simulink model "ModifiedHVDC"  (R2024b)
settings: Solver=ode3  StartTime=0.0  StopTime=2.5  FixedStep=7.4074074074074075E-6  RelTol=1e-3  AbsTol=1e-2
InitFcn:
  | Fnom = 50;        % Hz
  | 
  | Fc = 27*Fnom;   % (Hz)
  | Ts_Power = 1/(Fc*100);
  | Ts_Control = Ts_Power*10;
values from neighbouring files (symbols this model uses):
  C_per_km = 2.3100e-007    (= 2.31e-07)    [Parameters.m]
  L_per_km = 1.5900e-004    (= 0.000159)    [Parameters.m]
  L_total = 75    [Parameters.m]
  R_per_km = 1.3900e-002    (= 0.0139)    [Parameters.m]
  x_fault = 13    [Parameters.m]
undefined symbols (not defined in the file or in its folder): D1, Delta, DiscIntNeverNeededParam, magnitude
libraries: spsSecondOrderFilterLib x20, spsSeriesRLCBranchLib x14, spsMeanVariableFrequencyLib x12, spsabctoAlphaBetaZeroLib x8, spsThreePhaseVIMeasurementLib x6, spsAlphaBetaZerotodq0Lib x6, spsPiSectionLineLib x4, spsCurrentMeasurementLib x4, spsThreePhaseHarmonicFilterLib x4, spsVoltageMeasurementLib x4, spsFirstOrderFilterLib x4, spsGroundLib x3
(part 4 of 5)

== system ModifiedHVDC/VSC Controller Station 2/Discrete VSC Controller /Outer Active-Reactive Power and Voltage Loop/Reactive_Power_Control ==
  note: Output is added to the regulator reference
      |  in order to maintain the AC voltage within
      |  minimum and maximum limits
  note: Reactive Power Control
  enable_control : Inport
  Qref : Inport  Port=2
  Q_meas : Inport  Port=3
  U_meas : Inport  Port=4
  "AC Voltage Control Override " : Subsystem  mask(Regulator with override functionality){max_in=U_max, min_in=U_min, Ki=Ki_rpc_vco, Kp=Kp_rpc_vco, IC_i=0, max_out_lim=max_rpc_vco, min_out_lim=min_rpc_vco, Ts=Ts_Control}
      mask prompts: max_in "Input upper range (pu):"; min_in "Input lower range (pu):"; Ki "Integrator gain (pu/s):"; Kp "Proportional gain:"; IC_i "Integrator initial condition (pu):"; max_out_lim "Output maximum limit (pu):"; min_out_lim "Output minimum limit (pu):"; Ts "Sample time: (s)"
      mask Display: disp('Override \nRegulator')
  Add : Sum
  Freeze_integrator : Subsystem
  Gain : Gain  Gain=-1
  Int_regulator (type 1) : Subsystem  mask(Feed forward integral regulator with anti-windup and freeze - type 1){max_i=max_i_rpc, min_i=min_i_rpc, Ki=Ki_rpc, IC_i=0, Kf=1.0, max_out=Q_max, min_out=Q_min, Ts=Ts_Control}
      mask prompts: max_i "Integrator maximum  limit (pu):"; min_i "Integrator minimum  limit (pu):"; Ki "Integrator gain (pu/s):"; IC_i "Integrator initial condition (pu):"; Kf "Feadback gain :"; max_out "Output maximum limit (pu):"; min_out "Output minimum limit (pu):"; Ts "Sample time: (s)"
      mask help:
      | The reference (input 1) is fed forward to the output. The integrator compensates for any steady-state error between the desired (input 1) and the measured value input 2). The error signal (input 1 - input 2) is integrated with dynamic limits (Integrator min and max limits). The integration can be frozen (stopped) when input 3 is TRUE.
      | A back-calculation anti-windup method discharges the integrator on block saturation (output min and max limits) using a feedback loop having a gain coefficient.
      mask Display: disp('Integral \n(Type 1)')
  Saturation : Saturate  UpperLimit=Q_max  LowerLimit=Q_min
      settings: AttributesFormatString=Min=%<LowerLimit>\nMax=%<UpperLimit>
  Qref_rpc : Outport  VectorParamsAs1DForOutWhenUnconnected=off
  wires:
  Gain/1 -> Add/1
  Add/1 -> Saturation/1
  "AC Voltage Control Override "/1(Out) -> Add/2
  Int_regulator (type 1)/1(Out) -> Gain/1
  U_meas/1 -> Freeze_integrator/1(U_meas), "AC Voltage Control Override "/1(In)
  Saturation/1 -> Qref_rpc/1
  Qref/1 -> Int_regulator (type 1)/1(Ord)
  Q_meas/1 -> Int_regulator (type 1)/2(Meas)
  enable_control/1 -> Int_regulator (type 1)/Enable, "AC Voltage Control Override "/Enable
  Freeze_integrator/1(Freeze) -> Int_regulator (type 1)/3(freeze)

== system ModifiedHVDC/VSC Controller Station 2/Discrete VSC Controller /PLL/Discrete PI Controller ==
  note: Pierre Giroux, Gilbert Sybille
      | Power System Simulation Laboratory
      | IREQ, Hydro-Quebc
  note: Discrete PID Controller
  Error : Inport  SampleTime=Ts
  Discrete-Time Integrator : DiscreteIntegrator  InitialCondition=Init  SampleTime=Ts  LimitOutput=on  UpperSaturationLimit=UpperLimit  LowerSaturationLimit=LowerLimit  ICPrevOutput=DiscIntNeverNeededParam  ICPrevScaledInput=DiscIntNeverNeededParam
  Kp4 : Gain  Gain=Kp  SaturateOnIntegerOverflow=on  SampleTime=Ts  OutDataTypeStr=Inherit: Same as input  ParamDataTypeStr=Inherit: Same as input
  Kp5 : Gain  Gain=Ki  SaturateOnIntegerOverflow=on  SampleTime=Ts  OutDataTypeStr=Inherit: Same as input  ParamDataTypeStr=Inherit: Same as input
  Saturation2 : Saturate  UpperLimit=UpperLimit  LowerLimit=LowerLimit  SampleTime=Ts
  Sum6 : Sum  InputSameDT=on  SaturateOnIntegerOverflow=on  SampleTime=Ts  OutDataTypeStr=Inherit: Same as first input
  Zero-Order Hold : ZeroOrderHold  SampleTime=Ts
  Out : Outport  SampleTime=Ts  InitialOutput=0  VectorParamsAs1DForOutWhenUnconnected=off
  wires:
  Error/1 -> Kp4/1, Kp5/1
  Sum6/1 -> Saturation2/1
  Kp5/1 -> Discrete-Time Integrator/1
  Kp4/1 -> Zero-Order Hold/1
  Discrete-Time Integrator/1 -> Sum6/2
  Saturation2/1 -> Out/1
  Zero-Order Hold/1 -> Sum6/1

== system ModifiedHVDC/VSC Controller Station 2/Discrete VSC Controller /PLL/Discrete Rate Limiter ==
  note: Delta(u)
  note: Beat Ronner
      | ABB Industrie AG
      | Turgi, Switzerland
  In : Inport
  Saturation : Saturate  UpperLimit=UpperLimit  LowerLimit=LowerLimit
  Sum : Sum  Inputs=|++  InputSameDT=on  SaturateOnIntegerOverflow=on  OutDataTypeStr=Inherit: Same as first input
  Sum1 : Sum  Inputs=|+-  InputSameDT=on  SaturateOnIntegerOverflow=on  OutDataTypeStr=Inherit: Same as first input
  Unit Delay : UnitDelay  InitialCondition=Vinit  SampleTime=Ts  HasFrameUpgradeWarning=on
  Out : Outport  VectorParamsAs1DForOutWhenUnconnected=off
  wires:
  In/1 -> Sum1/1  "u"
  Sum1/1 -> Saturation/1
  Saturation/1 -> Sum/1  "Delta(u)_limit"
  Sum/1 -> Out/1, Unit Delay/1  "y"
  Unit Delay/1 -> Sum1/2, Sum/2  "y-1"

== system ModifiedHVDC/VSC Controller Station 2/Discrete VSC Controller /Signal Calculations/Active_Power ==
  note: Active Power Calculation
  U_AB : Inport
  I_AB : Inport  Port=2
  Demux : Demux  Outputs=2
      settings: DisplayOption=none
  Demux1 : Demux  Outputs=2
      settings: DisplayOption=none
  Product : Product  SaturateOnIntegerOverflow=on  OutDataTypeStr=Inherit: Same as first input
  Product1 : Product  SaturateOnIntegerOverflow=on  OutDataTypeStr=Inherit: Same as first input
  Sum : Sum  SaturateOnIntegerOverflow=on
  Ppcc : Outport  VectorParamsAs1DForOutWhenUnconnected=off
  wires:
  U_AB/1 -> Demux/1
  I_AB/1 -> Demux1/1
  Demux/1 -> Product/1
  Demux1/1 -> Product/2
  Demux/2 -> Product1/1
  Demux1/2 -> Product1/2
  Product/1 -> Sum/1
  Product1/1 -> Sum/2
  Sum/1 -> Ppcc/1

== system ModifiedHVDC/VSC Controller Station 2/Discrete VSC Controller /Signal Calculations/DC_Current ==
  note: DC Current Calculation
  Idc_p : Inport
  Idc_n : Inport  Port=2
  Gain : Gain  Gain=0.5  SaturateOnIntegerOverflow=on  OutDataTypeStr=Inherit: Same as input  ParamDataTypeStr=Inherit: Same as input
  Sum : Sum  Inputs=+-  SaturateOnIntegerOverflow=on
  Idc_meas : Outport  VectorParamsAs1DForOutWhenUnconnected=off
  wires:
  Gain/1 -> Idc_meas/1
  Sum/1 -> Gain/1
  Idc_n/1 -> Sum/2
  Idc_p/1 -> Sum/1

== system ModifiedHVDC/VSC Controller Station 2/Discrete VSC Controller /Signal Calculations/DC_Voltage ==
  note: DC Voltage Calculation
  Udc_p : Inport
  Udc_n : Inport  Port=2
  Gain : Gain  Gain=0.5  SaturateOnIntegerOverflow=on  OutDataTypeStr=Inherit: Same as input  ParamDataTypeStr=Inherit: Same as input
  Sum : Sum  Inputs=+-  SaturateOnIntegerOverflow=on
  Udc_meas : Outport  VectorParamsAs1DForOutWhenUnconnected=off
  wires:
  Udc_p/1 -> Sum/1
  Sum/1 -> Gain/1
  Gain/1 -> Udc_meas/1
  Udc_n/1 -> Sum/2

== system ModifiedHVDC/VSC Controller Station 2/Discrete VSC Controller /Signal Calculations/Filter_Bus_Voltage ==
  note: Filter Bus Voltage Calculation
  Uf_AB : Inport
  Math Function : Math  Operator=magnitude^2  SignedPower=on
  Math Function1 : Math  Operator=sqrt  SignedPower=on
  Sum : Sum  Inputs=+  SaturateOnIntegerOverflow=on
  Uf_meas : Outport  VectorParamsAs1DForOutWhenUnconnected=off
  wires:
  Math Function1/1 -> Uf_meas/1
  Sum/1 -> Math Function1/1
  Math Function/1 -> Sum/1
  Uf_AB/1 -> Math Function/1

== system ModifiedHVDC/VSC Controller Station 2/Discrete VSC Controller /Signal Calculations/Modulation_Index ==
  note: Modulation Index Calculation
  Vref_lim_AB : Inport
  Udc_meas : Inport  Port=2
  Gain1 : Gain  Gain=k_pu2nom_Vdc  SaturateOnIntegerOverflow=on  OutDataTypeStr=Inherit: Same as input  ParamDataTypeStr=Inherit: Same as input
  MAX:10 MIN: 0 : Saturate  UpperLimit=10  LowerLimit=0
  Math Function1 : Math  Operator=magnitude^2  SignedPower=on
  Math Function2 : Math  Operator=sqrt  SignedPower=on
  Product : Product  Inputs=*/  SaturateOnIntegerOverflow=on  OutDataTypeStr=Inherit: Same as first input
  Saturation : Saturate  UpperLimit=1e6  LowerLimit=1e-6
  Sum : Sum  Inputs=+  SaturateOnIntegerOverflow=on
  Mod_index : Outport  VectorParamsAs1DForOutWhenUnconnected=off
  wires:
  Gain1/1 -> Saturation/1
  MAX:10 MIN: 0/1 -> Mod_index/1
  Saturation/1 -> Product/2
  Product/1 -> MAX:10 MIN: 0/1
  Udc_meas/1 -> Gain1/1
  Sum/1 -> Math Function2/1
  Math Function1/1 -> Sum/1
  Math Function2/1 -> Product/1
  Vref_lim_AB/1 -> Math Function1/1

== system ModifiedHVDC/VSC Controller Station 2/Discrete VSC Controller /Signal Calculations/PCC_Voltage ==
  note: Active Power Calculation
  U_AB : Inport
  Math Function : Math  Operator=magnitude^2  SignedPower=on
  Math Function1 : Math  Operator=sqrt  SignedPower=on
  Sum : Sum  Inputs=+  SaturateOnIntegerOverflow=on
  Upcc : Outport  VectorParamsAs1DForOutWhenUnconnected=off
  wires:
  U_AB/1 -> Math Function/1
  Math Function/1 -> Sum/1
  Sum/1 -> Math Function1/1
  Math Function1/1 -> Upcc/1

== system ModifiedHVDC/VSC Controller Station 2/Discrete VSC Controller /Signal Calculations/Reactive_Power ==
  note: Reactive Power Calculation
  U_AB : Inport
  I_AB : Inport  Port=2
  Demux : Demux  Outputs=2
      settings: DisplayOption=none
  Demux1 : Demux  Outputs=2
      settings: DisplayOption=none
  Product : Product  SaturateOnIntegerOverflow=on  OutDataTypeStr=Inherit: Same as first input
  Product1 : Product  SaturateOnIntegerOverflow=on  OutDataTypeStr=Inherit: Same as first input
  Sum : Sum  Inputs=+-  SaturateOnIntegerOverflow=on
  Qpcc : Outport  VectorParamsAs1DForOutWhenUnconnected=off
  wires:
  Sum/1 -> Qpcc/1
  Product1/1 -> Sum/2
  Product/1 -> Sum/1
  I_AB/1 -> Demux1/1
  U_AB/1 -> Demux/1
  Demux/2 -> Product/2
  Demux1/1 -> Product/1
  Demux/1 -> Product1/1
  Demux1/2 -> Product1/2

== system ModifiedHVDC/VSC Controller Station 1/Discrete VSC Controller /Clark Transformations/CLARK  with Rotating reference/CLARK ==
  note: CLARK transformation
  abc : Inport
  Enable (held) : EnablePort  PropagateVarSize=During execution
  abc to Alpha-Beta-Zero : spsabctoAlphaBetaZeroLib/abc to Alpha-Beta-Zero
  AB0 : Outport  VectorParamsAs1DForOutWhenUnconnected=off
  wires:
  abc to Alpha-Beta-Zero/1 -> AB0/1
  abc/1 -> abc to Alpha-Beta-Zero/1

== system ModifiedHVDC/VSC Controller Station 1/Discrete VSC Controller /Clark Transformations/CLARK  with Rotating reference/CLARK_lag ==
  note: CLARK transformation - YD1
  abc : Inport
  Enable : EnablePort  PropagateVarSize=During execution
  Fcn1 : Fcn  Expr=(-u[1] - u[3] + 2*u[2] )/3
  Fcn2 : Fcn  Expr=(u[1]-u[3])/sqrt(3)
  Fcn3 : Fcn  Expr=0
  Mux : Mux  Inputs=3
  AB0 : Outport  VectorParamsAs1DForOutWhenUnconnected=off
  wires:
  Fcn2/1 -> Mux/1
  abc/1 -> Fcn1/1, Fcn3/1, Fcn2/1
  Fcn1/1 -> Mux/2
  Fcn3/1 -> Mux/3
  Mux/1 -> AB0/1

== system ModifiedHVDC/VSC Controller Station 1/Discrete VSC Controller /Clark Transformations/CLARK  with Rotating reference/CLARK_lead ==
  note: CLARK transformation - YD11
  abc : Inport
  Enable : EnablePort  PropagateVarSize=During execution
  Fcn1 : Fcn  Expr=(u[1] + u[2] - 2*u[3] )/3
  Fcn2 : Fcn  Expr=(u[1]-u[2])/sqrt(3)
  Fcn3 : Fcn  Expr=0
  Mux : Mux  Inputs=3
  AB0 : Outport  VectorParamsAs1DForOutWhenUnconnected=off
  wires:
  Mux/1 -> AB0/1
  Fcn3/1 -> Mux/3
  Fcn1/1 -> Mux/2
  abc/1 -> Fcn2/1, Fcn3/1, Fcn1/1
  Fcn2/1 -> Mux/1

== system ModifiedHVDC/VSC Controller Station 1/Discrete VSC Controller /Clark Transformations/CLARK  with Rotating reference1/CLARK ==
  note: CLARK transformation
  abc : Inport
  Enable (held) : EnablePort  PropagateVarSize=During execution
  abc to Alpha-Beta-Zero : spsabctoAlphaBetaZeroLib/abc to Alpha-Beta-Zero
  AB0 : Outport  VectorParamsAs1DForOutWhenUnconnected=off
  wires:
  abc to Alpha-Beta-Zero/1 -> AB0/1
  abc/1 -> abc to Alpha-Beta-Zero/1

== system ModifiedHVDC/VSC Controller Station 1/Discrete VSC Controller /Clark Transformations/CLARK  with Rotating reference1/CLARK_lag ==
  note: CLARK transformation - YD1
  abc : Inport
  Enable : EnablePort  PropagateVarSize=During execution
  Fcn1 : Fcn  Expr=(-u[1] - u[3] + 2*u[2] )/3
  Fcn2 : Fcn  Expr=(u[1]-u[3])/sqrt(3)
  Fcn3 : Fcn  Expr=0
  Mux : Mux  Inputs=3
  AB0 : Outport  VectorParamsAs1DForOutWhenUnconnected=off
  wires:
  Fcn2/1 -> Mux/1
  abc/1 -> Fcn1/1, Fcn3/1, Fcn2/1
  Fcn1/1 -> Mux/2
  Fcn3/1 -> Mux/3
  Mux/1 -> AB0/1

== system ModifiedHVDC/VSC Controller Station 1/Discrete VSC Controller /Clark Transformations/CLARK  with Rotating reference1/CLARK_lead ==
  note: CLARK transformation - YD11
  abc : Inport
  Enable : EnablePort  PropagateVarSize=During execution
  Fcn1 : Fcn  Expr=(u[1] + u[2] - 2*u[3] )/3
  Fcn2 : Fcn  Expr=(u[1]-u[2])/sqrt(3)
  Fcn3 : Fcn  Expr=0
  Mux : Mux  Inputs=3
  AB0 : Outport  VectorParamsAs1DForOutWhenUnconnected=off
  wires:
  Mux/1 -> AB0/1
  Fcn3/1 -> Mux/3
  Fcn1/1 -> Mux/2
  abc/1 -> Fcn2/1, Fcn3/1, Fcn1/1
  Fcn2/1 -> Mux/1

== system ModifiedHVDC/VSC Controller Station 1/Discrete VSC Controller /DC Voltage Balance Control/Regulator/PI_regulator (type 2) ==
  note: Regulator PI
      | (Type 2)
  Ord : Inport
  Meas : Inport  Port=2
  Add : Sum
  Add1 : Sum
  Discrete-Time Integrator : DiscreteIntegrator  IntegratorMethod=Integration: Trapezoidal  gainval=Ki  InitialCondition=i_ic  SampleTime=Ts  LimitOutput=on  UpperSaturationLimit=max_i  LowerSaturationLimit=min_i  ICPrevOutput=DiscIntNeverNeededParam  ICPrevScaledInput=DiscIntNeverNeededParam
      settings: AttributesFormatString=Gain=%<gainval>\nMin=%<LowerSaturationLimit>\nMax=%<UpperSaturationLimit>
  Kf : Gain  Gain=Kf
      settings: AttributesFormatString=Gain=%<Gain>
  Kp : Gain  Gain=Kp
      settings: AttributesFormatString=Gain=%<Gain>
  Saturation : Saturate  UpperLimit=max_out  LowerLimit=min_out
      settings: AttributesFormatString=Min=%<LowerLimit>\nMax=%<UpperLimit>
  Subtract : Sum  Inputs=+-
  Sum2 : Sum  Inputs=|+-  SaturateOnIntegerOverflow=on
  Unit Delay : UnitDelay  SampleTime=Ts_Control  HasFrameUpgradeWarning=on
      settings: AttributesFormatString=IC=%<InitialCondition>
  Out : Outport  VectorParamsAs1DForOutWhenUnconnected=off
  wires:
  Kp/1 -> Add1/1
  Sum2/1 -> Kf/1
  Subtract/1 -> Add/1, Kp/1
  Saturation/1 -> Sum2/1, Out/1
  Unit Delay/1 -> Add/2
  Add/1 -> Discrete-Time Integrator/1
  Ord/1 -> Subtract/1
  Kf/1 -> Unit Delay/1
  Add1/1 -> Saturation/1, Sum2/2
  Discrete-Time Integrator/1 -> Add1/2
  Meas/1 -> Subtract/2

== system ModifiedHVDC/VSC Controller Station 1/Discrete VSC Controller /Inner Current Loop/AC_Current_Control/PI_regulator 1 ==
  note: Regulator PI
      | (Type 2)
  Ord : Inport
  Meas : Inport  Port=2
  Add : Sum
  Add1 : Sum
  Discrete-Time Integrator : DiscreteIntegrator  IntegratorMethod=Integration: Trapezoidal  gainval=Ki  InitialCondition=i_ic  SampleTime=Ts  LimitOutput=on  UpperSaturationLimit=max_i  LowerSaturationLimit=min_i  ICPrevOutput=DiscIntNeverNeededParam  ICPrevScaledInput=DiscIntNeverNeededParam
      settings: AttributesFormatString=Gain=%<gainval>\nMin=%<LowerSaturationLimit>\nMax=%<UpperSaturationLimit>
  Kf : Gain  Gain=Kf
      settings: AttributesFormatString=Gain=%<Gain>
  Kp : Gain  Gain=Kp
      settings: AttributesFormatString=Gain=%<Gain>
  Saturation : Saturate  UpperLimit=max_out  LowerLimit=min_out
      settings: AttributesFormatString=Min=%<LowerLimit>\nMax=%<UpperLimit>
  Subtract : Sum  Inputs=+-
  Sum2 : Sum  Inputs=|+-  SaturateOnIntegerOverflow=on
  Unit Delay : UnitDelay  SampleTime=Ts_Control  HasFrameUpgradeWarning=on
      settings: AttributesFormatString=IC=%<InitialCondition>
  Out : Outport  VectorParamsAs1DForOutWhenUnconnected=off
  wires:
  Kp/1 -> Add1/1
  Sum2/1 -> Kf/1
  Subtract/1 -> Add/1, Kp/1
  Saturation/1 -> Sum2/1, Out/1
  Unit Delay/1 -> Add/2
  Add/1 -> Discrete-Time Integrator/1
  Ord/1 -> Subtract/1
  Kf/1 -> Unit Delay/1
  Add1/1 -> Saturation/1, Sum2/2
  Discrete-Time Integrator/1 -> Add1/2
  Meas/1 -> Subtract/2

== system ModifiedHVDC/VSC Controller Station 1/Discrete VSC Controller /Inner Current Loop/AC_Current_Control/PI_regulator 2 ==
  note: Regulator PI
      | (Type 2)
  Ord : Inport
  Meas : Inport  Port=2
  Add : Sum
  Add1 : Sum
  Discrete-Time Integrator : DiscreteIntegrator  IntegratorMethod=Integration: Trapezoidal  gainval=Ki  InitialCondition=i_ic  SampleTime=Ts  LimitOutput=on  UpperSaturationLimit=max_i  LowerSaturationLimit=min_i  ICPrevOutput=DiscIntNeverNeededParam  ICPrevScaledInput=DiscIntNeverNeededParam
      settings: AttributesFormatString=Gain=%<gainval>\nMin=%<LowerSaturationLimit>\nMax=%<UpperSaturationLimit>
  Kf : Gain  Gain=Kf
      settings: AttributesFormatString=Gain=%<Gain>
  Kp : Gain  Gain=Kp
      settings: AttributesFormatString=Gain=%<Gain>
  Saturation : Saturate  UpperLimit=max_out  LowerLimit=min_out
      settings: AttributesFormatString=Min=%<LowerLimit>\nMax=%<UpperLimit>
  Subtract : Sum  Inputs=+-
  Sum2 : Sum  Inputs=|+-  SaturateOnIntegerOverflow=on
  Unit Delay : UnitDelay  SampleTime=Ts_Control  HasFrameUpgradeWarning=on
      settings: AttributesFormatString=IC=%<InitialCondition>
  Out : Outport  VectorParamsAs1DForOutWhenUnconnected=off
  wires:
  Kp/1 -> Add1/1
  Sum2/1 -> Kf/1
  Subtract/1 -> Add/1, Kp/1
  Saturation/1 -> Sum2/1, Out/1
  Unit Delay/1 -> Add/2
  Add/1 -> Discrete-Time Integrator/1
  Ord/1 -> Subtract/1
  Kf/1 -> Unit Delay/1
  Add1/1 -> Saturation/1, Sum2/2
  Discrete-Time Integrator/1 -> Add1/2
  Meas/1 -> Subtract/2

== system ModifiedHVDC/VSC Controller Station 1/Discrete VSC Controller /Outer Active-Reactive Power and Voltage Loop/Active_Power_Control/DC Voltage Control Override ==
  note: Reset states when enabling
  note: Override Regulator
  note: Active when input (In) is outside its range [min_in, max_in] otherwise the output goes back to zero
  In : Inport
  Enable (reset) : EnablePort  StatesWhenEnabling=reset  PropagateVarSize=During execution
  Add : Sum
  Constant1 : Constant  Value=max_in
  Constant2 : Constant  Value=min_in
  Constant3 : Constant  Value=Kp
  Discrete-Time Integrator1 : DiscreteIntegrator  IntegratorMethod=Integration: Trapezoidal  gainval=Ki  InitialCondition=IC_i  SampleTime=Ts  LimitOutput=on  UpperSaturationLimit=0  LowerSaturationLimit=min_out_lim  ICPrevOutput=DiscIntNeverNeededParam  ICPrevScaledInput=DiscIntNeverNeededParam
      settings: AttributesFormatString=Gain=%<gainval>\nMin=%<LowerSaturationLimit>\nMax=%<UpperSaturationLimit>
  Discrete-Time Integrator2 : DiscreteIntegrator  IntegratorMethod=Integration: Trapezoidal  gainval=Ki  InitialCondition=IC_i  SampleTime=Ts  LimitOutput=on  UpperSaturationLimit=max_out_lim  LowerSaturationLimit=0  ICPrevOutput=DiscIntNeverNeededParam  ICPrevScaledInput=DiscIntNeverNeededParam
      settings: AttributesFormatString=Gain=%<gainval>\nMin=%<LowerSaturationLimit>\nMax=%<UpperSaturationLimit>
  Product : Product  RndMeth=Zero
  Saturation : Saturate  UpperLimit=0  LowerLimit=min_out_lim
      settings: AttributesFormatString=Min=%<LowerLimit>\nMax=%<UpperLimit>
  Saturation1 : Saturate  UpperLimit=max_out_lim  LowerLimit=0
      settings: AttributesFormatString=Min=%<LowerLimit>\nMax=%<UpperLimit>
  Saturation2 : Saturate  UpperLimit=max_out_lim  LowerLimit=min_out_lim
      settings: AttributesFormatString=Min=%<LowerLimit>\nMax=%<UpperLimit>
  Subtract : Sum  Inputs=+-
  Subtract1 : Sum  Inputs=-+
  Sum2 : Sum  Inputs=+++  SaturateOnIntegerOverflow=on
  Out : Outport  VectorParamsAs1DForOutWhenUnconnected=off
  wires:
  Constant2/1 -> Subtract1/2
  Constant1/1 -> Subtract/1
  Discrete-Time Integrator2/1 -> Sum2/3  "positive"
  Discrete-Time Integrator1/1 -> Sum2/2  "negative"
  Product/1 -> Sum2/1
  Saturation1/1 -> Add/2
  Saturation/1 -> Add/1
  Add/1 -> Product/2
  Constant3/1 -> Product/1
  In/1 -> Subtract1/1, Subtract/2
  Subtract/1 -> Discrete-Time Integrator1/1, Saturation/1
  Subtract1/1 -> Saturation1/1, Discrete-Time Integrator2/1
  Sum2/1 -> Saturation2/1
  Saturation2/1 -> Out/1

== system ModifiedHVDC/VSC Controller Station 1/Discrete VSC Controller /Outer Active-Reactive Power and Voltage Loop/Active_Power_Control/Freeze_integrator ==
  note: Low AC voltage level
  note: Freeze Integrator
  U_meas : Inport
  Constant8 : Constant  Value=V_level_apc
  Relational Operator : RelationalOperator  Operator=<=  InputSameDT=off
  Freeze : Outport  VectorParamsAs1DForOutWhenUnconnected=off
  wires:
  Constant8/1 -> Relational Operator/2
  Relational Operator/1 -> Freeze/1
  U_meas/1 -> Relational Operator/1

== system ModifiedHVDC/VSC Controller Station 1/Discrete VSC Controller /Outer Active-Reactive Power and Voltage Loop/Active_Power_Control/Int_regulator (type 1) ==
  note: Reset states when enabling
  note: Integral Regulator
      | (Type 1)
  Ord : Inport
  Meas : Inport  Port=2
  freeze : Inport  Port=3
  Enable (Reset) : EnablePort  StatesWhenEnabling=reset  PropagateVarSize=During execution
  Add : Sum
  Add1 : Sum
  Constant7 : Constant  Value=0.0
  Discrete-Time Integrator : DiscreteIntegrator  IntegratorMethod=Integration: Trapezoidal  gainval=Ki  InitialCondition=IC_i  SampleTime=Ts  LimitOutput=on  UpperSaturationLimit=max_i  LowerSaturationLimit=min_i  ICPrevOutput=DiscIntNeverNeededParam  ICPrevScaledInput=DiscIntNeverNeededParam
      settings: AttributesFormatString=Gain=%<gainval>\nMin=%<LowerSaturationLimit>\nMax=%<UpperSaturationLimit>
  Kf : Gain  Gain=Kf
      settings: AttributesFormatString=Gain=%<Gain>
  Saturation : Saturate  UpperLimit=max_out  LowerLimit=min_out
      settings: AttributesFormatString=Min=%<LowerLimit>\nMax=%<UpperLimit>
  Subtract : Sum  Inputs=+-
  Sum2 : Sum  Inputs=|+-  SaturateOnIntegerOverflow=on
  Switch : Switch  Criteria=u2 > Threshold  InputSameDT=off
  Unit Delay : UnitDelay  SampleTime=Ts_Control  HasFrameUpgradeWarning=on
      settings: AttributesFormatString=IC=%<InitialCondition>
  Out : Outport  VectorParamsAs1DForOutWhenUnconnected=off
  wires:
  Kf/1 -> Unit Delay/1
  Subtract/1 -> Switch/3
  Meas/1 -> Subtract/2
  Switch/1 -> Add/1
  Constant7/1 -> Switch/1
  freeze/1 -> Switch/2
  Discrete-Time Integrator/1 -> Add1/2
  Add1/1 -> Sum2/2, Saturation/1
  Sum2/1 -> Kf/1
  Ord/1 -> Subtract/1, Add1/1
  Add/1 -> Discrete-Time Integrator/1
  Unit Delay/1 -> Add/2
  Saturation/1 -> Sum2/1, Out/1

== system ModifiedHVDC/VSC Controller Station 1/Discrete VSC Controller /Outer Active-Reactive Power and Voltage Loop/Active_Power_Control/Ramping ==
  note: Output is reset to zero when the ramp is not enabled
  note: Ramping
  enable_ramp : Inport
  Pref : Inport  Port=2
  Constant12 : Constant  Value=Ramp_apc
  Logical Operator7 : Logic  Operator=NOT  AllPortsSameDT=off
  Rate Limiter with external rates & reset (discrete) IC:0 : Subsystem  mask(Rate of Change Limiter){ic=0, st=Ts_Control}
      mask prompts: ic "Initial condition (pu):"; st "Sample time (s):"
      mask help: Limit rising and falling rates of signal. When the input (R) is true the output is reset to the input (In). Rates are in p.u./s for up and -p.u./s for down.
      mask Display: disp('                Rate\n               Limiter')
  Switch : Switch  Criteria=u2 > Threshold  InputSameDT=off
  zero : Constant  Value=0.0
  Pref_ramp : Outport  VectorParamsAs1DForOutWhenUnconnected=off
  wires:
  Logical Operator7/1 -> Rate Limiter with external rates & reset (discrete) IC:0/4(R)
  Switch/1 -> Rate Limiter with external rates & reset (discrete) IC:0/1(In)
  zero/1 -> Switch/3
  Pref/1 -> Switch/1
  enable_ramp/1 -> Logical Operator7/1, Switch/2
  Constant12/1 -> Rate Limiter with external rates & reset (discrete) IC:0/3(down_rate), Rate Limiter with external rates & reset (discrete) IC:0/2(up_rate)
  Rate Limiter with external rates & reset (discrete) IC:0/1(" ") -> Pref_ramp/1

== system ModifiedHVDC/VSC Controller Station 1/Discrete VSC Controller /Outer Active-Reactive Power and Voltage Loop/Current_Reference_Limitation/Double click here for  info ==
  note: Power System Simulation laboratory (IREQ)
  note: Current Reference Limitation
  note: The subsystem limits the amplitude of phase current of the fundamental component to the rated current
      | of the converter.
  note: Power Control Mode
  note: DC Voltage Control Mode
  note: In power control mode, equal scaling is applied to the active and reactive power reference when a limit is imposed.
  note: In DC voltage control mode, higher priority is given to the active power when a limit is imposed.

== system ModifiedHVDC/VSC Controller Station 1/Discrete VSC Controller /Outer Active-Reactive Power and Voltage Loop/DC_Voltage_Control/PI_regulator (type 2) ==
  note: Regulator PI
      | (Type 2)
  Ord : Inport
  Meas : Inport  Port=2
  Add : Sum
  Add1 : Sum
  Discrete-Time Integrator : DiscreteIntegrator  IntegratorMethod=Integration: Trapezoidal  gainval=Ki  InitialCondition=i_ic  SampleTime=Ts  LimitOutput=on  UpperSaturationLimit=max_i  LowerSaturationLimit=min_i  ICPrevOutput=DiscIntNeverNeededParam  ICPrevScaledInput=DiscIntNeverNeededParam
      settings: AttributesFormatString=Gain=%<gainval>\nMin=%<LowerSaturationLimit>\nMax=%<UpperSaturationLimit>
  Kf : Gain  Gain=Kf
      settings: AttributesFormatString=Gain=%<Gain>
  Kp : Gain  Gain=Kp
      settings: AttributesFormatString=Gain=%<Gain>
  Saturation : Saturate  UpperLimit=max_out  LowerLimit=min_out
      settings: AttributesFormatString=Min=%<LowerLimit>\nMax=%<UpperLimit>
  Subtract : Sum  Inputs=+-
  Sum2 : Sum  Inputs=|+-  SaturateOnIntegerOverflow=on
  Unit Delay : UnitDelay  SampleTime=Ts_Control  HasFrameUpgradeWarning=on
      settings: AttributesFormatString=IC=%<InitialCondition>
  Out : Outport  VectorParamsAs1DForOutWhenUnconnected=off
  wires:
  Kp/1 -> Add1/1
  Sum2/1 -> Kf/1
  Subtract/1 -> Add/1, Kp/1
  Saturation/1 -> Sum2/1, Out/1
  Unit Delay/1 -> Add/2
  Add/1 -> Discrete-Time Integrator/1
  Ord/1 -> Subtract/1
  Kf/1 -> Unit Delay/1
  Add1/1 -> Saturation/1, Sum2/2
  Discrete-Time Integrator/1 -> Add1/2
  Meas/1 -> Subtract/2

== system ModifiedHVDC/VSC Controller Station 1/Discrete VSC Controller /Outer Active-Reactive Power and Voltage Loop/Reactive_Power_Control/AC Voltage Control Override  ==
  note: Reset states when enabling
  note: Override Regulator
  note: Active when input (In) is outside its range [min_in, max_in] otherwise the output goes back to zero
  In : Inport
  Enable (reset) : EnablePort  StatesWhenEnabling=reset  PropagateVarSize=During execution
  Add : Sum
  Constant1 : Constant  Value=max_in
  Constant2 : Constant  Value=min_in
  Constant3 : Constant  Value=Kp
  Discrete-Time Integrator1 : DiscreteIntegrator  IntegratorMethod=Integration: Trapezoidal  gainval=Ki  InitialCondition=IC_i  SampleTime=Ts  LimitOutput=on  UpperSaturationLimit=0  LowerSaturationLimit=min_out_lim  ICPrevOutput=DiscIntNeverNeededParam  ICPrevScaledInput=DiscIntNeverNeededParam
      settings: AttributesFormatString=Gain=%<gainval>\nMin=%<LowerSaturationLimit>\nMax=%<UpperSaturationLimit>
  Discrete-Time Integrator2 : DiscreteIntegrator  IntegratorMethod=Integration: Trapezoidal  gainval=Ki  InitialCondition=IC_i  SampleTime=Ts  LimitOutput=on  UpperSaturationLimit=max_out_lim  LowerSaturationLimit=0  ICPrevOutput=DiscIntNeverNeededParam  ICPrevScaledInput=DiscIntNeverNeededParam
      settings: AttributesFormatString=Gain=%<gainval>\nMin=%<LowerSaturationLimit>\nMax=%<UpperSaturationLimit>
  Product : Product  RndMeth=Zero
  Saturation : Saturate  UpperLimit=0  LowerLimit=min_out_lim
      settings: AttributesFormatString=Min=%<LowerLimit>\nMax=%<UpperLimit>
  Saturation1 : Saturate  UpperLimit=max_out_lim  LowerLimit=0
      settings: AttributesFormatString=Min=%<LowerLimit>\nMax=%<UpperLimit>
  Saturation2 : Saturate  UpperLimit=max_out_lim  LowerLimit=min_out_lim
      settings: AttributesFormatString=Min=%<LowerLimit>\nMax=%<UpperLimit>
  Subtract : Sum  Inputs=+-
  Subtract1 : Sum  Inputs=-+
  Sum2 : Sum  Inputs=+++  SaturateOnIntegerOverflow=on
  Out : Outport  VectorParamsAs1DForOutWhenUnconnected=off
  wires:
  Constant2/1 -> Subtract1/2
  Constant1/1 -> Subtract/1
  Discrete-Time Integrator2/1 -> Sum2/3  "positive"
  Discrete-Time Integrator1/1 -> Sum2/2  "negative"
  Product/1 -> Sum2/1
  Saturation1/1 -> Add/2
  Saturation/1 -> Add/1
  Add/1 -> Product/2
  Constant3/1 -> Product/1
  In/1 -> Subtract1/1, Subtract/2
  Subtract/1 -> Discrete-Time Integrator1/1, Saturation/1
  Subtract1/1 -> Saturation1/1, Discrete-Time Integrator2/1
  Sum2/1 -> Saturation2/1
  Saturation2/1 -> Out/1

== system ModifiedHVDC/VSC Controller Station 1/Discrete VSC Controller /Outer Active-Reactive Power and Voltage Loop/Reactive_Power_Control/Freeze_integrator ==
  note: Freeze Integrator
  note: Low AC voltage level
  U_meas : Inport
  Constant8 : Constant  Value=V_level_rpc
  Relational Operator : RelationalOperator  Operator=<=  InputSameDT=off
  Freeze : Outport  VectorParamsAs1DForOutWhenUnconnected=off
  wires:
  U_meas/1 -> Relational Operator/1
  Relational Operator/1 -> Freeze/1
  Constant8/1 -> Relational Operator/2

== system ModifiedHVDC/VSC Controller Station 1/Discrete VSC Controller /Outer Active-Reactive Power and Voltage Loop/Reactive_Power_Control/Int_regulator (type 1) ==
  note: Reset states when enabling
  note: Integral Regulator
      | (Type 1)
  Ord : Inport
  Meas : Inport  Port=2
  freeze : Inport  Port=3
  Enable (Reset) : EnablePort  StatesWhenEnabling=reset  PropagateVarSize=During execution
  Add : Sum
  Add1 : Sum
  Constant7 : Constant  Value=0.0
  Discrete-Time Integrator : DiscreteIntegrator  IntegratorMethod=Integration: Trapezoidal  gainval=Ki  InitialCondition=IC_i  SampleTime=Ts  LimitOutput=on  UpperSaturationLimit=max_i  LowerSaturationLimit=min_i  ICPrevOutput=DiscIntNeverNeededParam  ICPrevScaledInput=DiscIntNeverNeededParam
      settings: AttributesFormatString=Gain=%<gainval>\nMin=%<LowerSaturationLimit>\nMax=%<UpperSaturationLimit>
  Kf : Gain  Gain=Kf
      settings: AttributesFormatString=Gain=%<Gain>
  Saturation : Saturate  UpperLimit=max_out  LowerLimit=min_out
      settings: AttributesFormatString=Min=%<LowerLimit>\nMax=%<UpperLimit>
  Subtract : Sum  Inputs=+-
  Sum2 : Sum  Inputs=|+-  SaturateOnIntegerOverflow=on
  Switch : Switch  Criteria=u2 > Threshold  InputSameDT=off
  Unit Delay : UnitDelay  SampleTime=Ts_Control  HasFrameUpgradeWarning=on
      settings: AttributesFormatString=IC=%<InitialCondition>
  Out : Outport  VectorParamsAs1DForOutWhenUnconnected=off
  wires:
  Kf/1 -> Unit Delay/1
  Subtract/1 -> Switch/3
  Meas/1 -> Subtract/2
  Switch/1 -> Add/1
  Constant7/1 -> Switch/1
  freeze/1 -> Switch/2
  Discrete-Time Integrator/1 -> Add1/2
  Add1/1 -> Sum2/2, Saturation/1
  Sum2/1 -> Kf/1
  Ord/1 -> Subtract/1, Add1/1
  Add/1 -> Discrete-Time Integrator/1
  Unit Delay/1 -> Add/2
  Saturation/1 -> Sum2/1, Out/1

== system ModifiedHVDC/VSC Controller Station 2/Discrete VSC Controller /Clark Transformations/CLARK  with Rotating reference/CLARK ==
  note: CLARK transformation
  abc : Inport
  Enable (held) : EnablePort  PropagateVarSize=During execution
  abc to Alpha-Beta-Zero : spsabctoAlphaBetaZeroLib/abc to Alpha-Beta-Zero
  AB0 : Outport  VectorParamsAs1DForOutWhenUnconnected=off
  wires:
  abc to Alpha-Beta-Zero/1 -> AB0/1
  abc/1 -> abc to Alpha-Beta-Zero/1

== system ModifiedHVDC/VSC Controller Station 2/Discrete VSC Controller /Clark Transformations/CLARK  with Rotating reference/CLARK_lag ==
  note: CLARK transformation - YD1
  abc : Inport
  Enable : EnablePort  PropagateVarSize=During execution
  Fcn1 : Fcn  Expr=(-u[1] - u[3] + 2*u[2] )/3
  Fcn2 : Fcn  Expr=(u[1]-u[3])/sqrt(3)
  Fcn3 : Fcn  Expr=0
  Mux : Mux  Inputs=3
  AB0 : Outport  VectorParamsAs1DForOutWhenUnconnected=off
  wires:
  Fcn2/1 -> Mux/1
  abc/1 -> Fcn1/1, Fcn3/1, Fcn2/1
  Fcn1/1 -> Mux/2
  Fcn3/1 -> Mux/3
  Mux/1 -> AB0/1

== system ModifiedHVDC/VSC Controller Station 2/Discrete VSC Controller /Clark Transformations/CLARK  with Rotating reference/CLARK_lead ==
  note: CLARK transformation - YD11
  abc : Inport
  Enable : EnablePort  PropagateVarSize=During execution
  Fcn1 : Fcn  Expr=(u[1] + u[2] - 2*u[3] )/3
  Fcn2 : Fcn  Expr=(u[1]-u[2])/sqrt(3)
  Fcn3 : Fcn  Expr=0
  Mux : Mux  Inputs=3
  AB0 : Outport  VectorParamsAs1DForOutWhenUnconnected=off
  wires:
  Mux/1 -> AB0/1
  Fcn3/1 -> Mux/3
  Fcn1/1 -> Mux/2
  abc/1 -> Fcn2/1, Fcn3/1, Fcn1/1
  Fcn2/1 -> Mux/1

== system ModifiedHVDC/VSC Controller Station 2/Discrete VSC Controller /Clark Transformations/CLARK  with Rotating reference1/CLARK ==
  note: CLARK transformation
  abc : Inport
  Enable (held) : EnablePort  PropagateVarSize=During execution
  abc to Alpha-Beta-Zero : spsabctoAlphaBetaZeroLib/abc to Alpha-Beta-Zero
  AB0 : Outport  VectorParamsAs1DForOutWhenUnconnected=off
  wires:
  abc to Alpha-Beta-Zero/1 -> AB0/1
  abc/1 -> abc to Alpha-Beta-Zero/1

== system ModifiedHVDC/VSC Controller Station 2/Discrete VSC Controller /Clark Transformations/CLARK  with Rotating reference1/CLARK_lag ==
  note: CLARK transformation - YD1
  abc : Inport
  Enable : EnablePort  PropagateVarSize=During execution
  Fcn1 : Fcn  Expr=(-u[1] - u[3] + 2*u[2] )/3
  Fcn2 : Fcn  Expr=(u[1]-u[3])/sqrt(3)
  Fcn3 : Fcn  Expr=0
  Mux : Mux  Inputs=3
  AB0 : Outport  VectorParamsAs1DForOutWhenUnconnected=off
  wires:
  Fcn2/1 -> Mux/1
  abc/1 -> Fcn1/1, Fcn3/1, Fcn2/1
  Fcn1/1 -> Mux/2
  Fcn3/1 -> Mux/3
  Mux/1 -> AB0/1

== system ModifiedHVDC/VSC Controller Station 2/Discrete VSC Controller /Clark Transformations/CLARK  with Rotating reference1/CLARK_lead ==
  note: CLARK transformation - YD11
  abc : Inport
  Enable : EnablePort  PropagateVarSize=During execution
  Fcn1 : Fcn  Expr=(u[1] + u[2] - 2*u[3] )/3
  Fcn2 : Fcn  Expr=(u[1]-u[2])/sqrt(3)
  Fcn3 : Fcn  Expr=0
  Mux : Mux  Inputs=3
  AB0 : Outport  VectorParamsAs1DForOutWhenUnconnected=off
  wires:
  Mux/1 -> AB0/1
  Fcn3/1 -> Mux/3
  Fcn1/1 -> Mux/2
  abc/1 -> Fcn2/1, Fcn3/1, Fcn1/1
  Fcn2/1 -> Mux/1

== system ModifiedHVDC/VSC Controller Station 2/Discrete VSC Controller /DC Voltage Balance Control/Regulator/PI_regulator (type 2) ==
  note: Regulator PI
      | (Type 2)
  Ord : Inport
  Meas : Inport  Port=2
  Add : Sum
  Add1 : Sum
  Discrete-Time Integrator : DiscreteIntegrator  IntegratorMethod=Integration: Trapezoidal  gainval=Ki  InitialCondition=i_ic  SampleTime=Ts  LimitOutput=on  UpperSaturationLimit=max_i  LowerSaturationLimit=min_i  ICPrevOutput=DiscIntNeverNeededParam  ICPrevScaledInput=DiscIntNeverNeededParam
      settings: AttributesFormatString=Gain=%<gainval>\nMin=%<LowerSaturationLimit>\nMax=%<UpperSaturationLimit>
  Kf : Gain  Gain=Kf
      settings: AttributesFormatString=Gain=%<Gain>
  Kp : Gain  Gain=Kp
      settings: AttributesFormatString=Gain=%<Gain>
  Saturation : Saturate  UpperLimit=max_out  LowerLimit=min_out
      settings: AttributesFormatString=Min=%<LowerLimit>\nMax=%<UpperLimit>
  Subtract : Sum  Inputs=+-
  Sum2 : Sum  Inputs=|+-  SaturateOnIntegerOverflow=on
  Unit Delay : UnitDelay  SampleTime=Ts_Control  HasFrameUpgradeWarning=on
      settings: AttributesFormatString=IC=%<InitialCondition>
  Out : Outport  VectorParamsAs1DForOutWhenUnconnected=off
  wires:
  Kp/1 -> Add1/1
  Sum2/1 -> Kf/1
  Subtract/1 -> Add/1, Kp/1
  Saturation/1 -> Sum2/1, Out/1
  Unit Delay/1 -> Add/2
  Add/1 -> Discrete-Time Integrator/1
  Ord/1 -> Subtract/1
  Kf/1 -> Unit Delay/1
  Add1/1 -> Saturation/1, Sum2/2
  Discrete-Time Integrator/1 -> Add1/2
  Meas/1 -> Subtract/2

== system ModifiedHVDC/VSC Controller Station 2/Discrete VSC Controller /Inner Current Loop/AC_Current_Control/PI_regulator 1 ==
  note: Regulator PI
      | (Type 2)
  Ord : Inport
  Meas : Inport  Port=2
  Add : Sum
  Add1 : Sum
  Discrete-Time Integrator : DiscreteIntegrator  IntegratorMethod=Integration: Trapezoidal  gainval=Ki  InitialCondition=i_ic  SampleTime=Ts  LimitOutput=on  UpperSaturationLimit=max_i  LowerSaturationLimit=min_i  ICPrevOutput=DiscIntNeverNeededParam  ICPrevScaledInput=DiscIntNeverNeededParam
      settings: AttributesFormatString=Gain=%<gainval>\nMin=%<LowerSaturationLimit>\nMax=%<UpperSaturationLimit>
  Kf : Gain  Gain=Kf
      settings: AttributesFormatString=Gain=%<Gain>
  Kp : Gain  Gain=Kp
      settings: AttributesFormatString=Gain=%<Gain>
  Saturation : Saturate  UpperLimit=max_out  LowerLimit=min_out
      settings: AttributesFormatString=Min=%<LowerLimit>\nMax=%<UpperLimit>
  Subtract : Sum  Inputs=+-
  Sum2 : Sum  Inputs=|+-  SaturateOnIntegerOverflow=on
  Unit Delay : UnitDelay  SampleTime=Ts_Control  HasFrameUpgradeWarning=on
      settings: AttributesFormatString=IC=%<InitialCondition>
  Out : Outport  VectorParamsAs1DForOutWhenUnconnected=off
  wires:
  Kp/1 -> Add1/1
  Sum2/1 -> Kf/1
  Subtract/1 -> Add/1, Kp/1
  Saturation/1 -> Sum2/1, Out/1
  Unit Delay/1 -> Add/2
  Add/1 -> Discrete-Time Integrator/1
  Ord/1 -> Subtract/1
  Kf/1 -> Unit Delay/1
  Add1/1 -> Saturation/1, Sum2/2
  Discrete-Time Integrator/1 -> Add1/2
  Meas/1 -> Subtract/2

== system ModifiedHVDC/VSC Controller Station 2/Discrete VSC Controller /Inner Current Loop/AC_Current_Control/PI_regulator 2 ==
  note: Regulator PI
      | (Type 2)
  Ord : Inport
  Meas : Inport  Port=2
  Add : Sum
  Add1 : Sum
  Discrete-Time Integrator : DiscreteIntegrator  IntegratorMethod=Integration: Trapezoidal  gainval=Ki  InitialCondition=i_ic  SampleTime=Ts  LimitOutput=on  UpperSaturationLimit=max_i  LowerSaturationLimit=min_i  ICPrevOutput=DiscIntNeverNeededParam  ICPrevScaledInput=DiscIntNeverNeededParam
      settings: AttributesFormatString=Gain=%<gainval>\nMin=%<LowerSaturationLimit>\nMax=%<UpperSaturationLimit>
  Kf : Gain  Gain=Kf
      settings: AttributesFormatString=Gain=%<Gain>
  Kp : Gain  Gain=Kp
      settings: AttributesFormatString=Gain=%<Gain>
  Saturation : Saturate  UpperLimit=max_out  LowerLimit=min_out
      settings: AttributesFormatString=Min=%<LowerLimit>\nMax=%<UpperLimit>
  Subtract : Sum  Inputs=+-
  Sum2 : Sum  Inputs=|+-  SaturateOnIntegerOverflow=on
  Unit Delay : UnitDelay  SampleTime=Ts_Control  HasFrameUpgradeWarning=on
      settings: AttributesFormatString=IC=%<InitialCondition>
  Out : Outport  VectorParamsAs1DForOutWhenUnconnected=off
  wires:
  Kp/1 -> Add1/1
  Sum2/1 -> Kf/1
  Subtract/1 -> Add/1, Kp/1
  Saturation/1 -> Sum2/1, Out/1
  Unit Delay/1 -> Add/2
  Add/1 -> Discrete-Time Integrator/1
  Ord/1 -> Subtract/1
  Kf/1 -> Unit Delay/1
  Add1/1 -> Saturation/1, Sum2/2
  Discrete-Time Integrator/1 -> Add1/2
  Meas/1 -> Subtract/2

== system ModifiedHVDC/VSC Controller Station 2/Discrete VSC Controller /Outer Active-Reactive Power and Voltage Loop/Active_Power_Control/DC Voltage Control Override ==
  note: Reset states when enabling
  note: Override Regulator
  note: Active when input (In) is outside its range [min_in, max_in] otherwise the output goes back to zero
  In : Inport
  Enable (reset) : EnablePort  StatesWhenEnabling=reset  PropagateVarSize=During execution
  Add : Sum
  Constant1 : Constant  Value=max_in
  Constant2 : Constant  Value=min_in
  Constant3 : Constant  Value=Kp
  Discrete-Time Integrator1 : DiscreteIntegrator  IntegratorMethod=Integration: Trapezoidal  gainval=Ki  InitialCondition=IC_i  SampleTime=Ts  LimitOutput=on  UpperSaturationLimit=0  LowerSaturationLimit=min_out_lim  ICPrevOutput=DiscIntNeverNeededParam  ICPrevScaledInput=DiscIntNeverNeededParam
      settings: AttributesFormatString=Gain=%<gainval>\nMin=%<LowerSaturationLimit>\nMax=%<UpperSaturationLimit>
  Discrete-Time Integrator2 : DiscreteIntegrator  IntegratorMethod=Integration: Trapezoidal  gainval=Ki  InitialCondition=IC_i  SampleTime=Ts  LimitOutput=on  UpperSaturationLimit=max_out_lim  LowerSaturationLimit=0  ICPrevOutput=DiscIntNeverNeededParam  ICPrevScaledInput=DiscIntNeverNeededParam
      settings: AttributesFormatString=Gain=%<gainval>\nMin=%<LowerSaturationLimit>\nMax=%<UpperSaturationLimit>
  Product : Product  RndMeth=Zero
  Saturation : Saturate  UpperLimit=0  LowerLimit=min_out_lim
      settings: AttributesFormatString=Min=%<LowerLimit>\nMax=%<UpperLimit>
  Saturation1 : Saturate  UpperLimit=max_out_lim  LowerLimit=0
      settings: AttributesFormatString=Min=%<LowerLimit>\nMax=%<UpperLimit>
  Saturation2 : Saturate  UpperLimit=max_out_lim  LowerLimit=min_out_lim
      settings: AttributesFormatString=Min=%<LowerLimit>\nMax=%<UpperLimit>
  Subtract : Sum  Inputs=+-
  Subtract1 : Sum  Inputs=-+
  Sum2 : Sum  Inputs=+++  SaturateOnIntegerOverflow=on
  Out : Outport  VectorParamsAs1DForOutWhenUnconnected=off
  wires:
  Constant2/1 -> Subtract1/2
  Constant1/1 -> Subtract/1
  Discrete-Time Integrator2/1 -> Sum2/3  "positive"
  Discrete-Time Integrator1/1 -> Sum2/2  "negative"
  Product/1 -> Sum2/1
  Saturation1/1 -> Add/2
  Saturation/1 -> Add/1
  Add/1 -> Product/2
  Constant3/1 -> Product/1
  In/1 -> Subtract1/1, Subtract/2
  Subtract/1 -> Discrete-Time Integrator1/1, Saturation/1
  Subtract1/1 -> Saturation1/1, Discrete-Time Integrator2/1
  Sum2/1 -> Saturation2/1
  Saturation2/1 -> Out/1

== system ModifiedHVDC/VSC Controller Station 2/Discrete VSC Controller /Outer Active-Reactive Power and Voltage Loop/Active_Power_Control/Freeze_integrator ==
  note: Low AC voltage level
  note: Freeze Integrator
  U_meas : Inport
  Constant8 : Constant  Value=V_level_apc
  Relational Operator : RelationalOperator  Operator=<=  InputSameDT=off
  Freeze : Outport  VectorParamsAs1DForOutWhenUnconnected=off
  wires:
  Constant8/1 -> Relational Operator/2
  Relational Operator/1 -> Freeze/1
  U_meas/1 -> Relational Operator/1

== system ModifiedHVDC/VSC Controller Station 2/Discrete VSC Controller /Outer Active-Reactive Power and Voltage Loop/Active_Power_Control/Int_regulator (type 1) ==
  note: Reset states when enabling
  note: Integral Regulator
      | (Type 1)
  Ord : Inport
  Meas : Inport  Port=2
  freeze : Inport  Port=3
  Enable (Reset) : EnablePort  StatesWhenEnabling=reset  PropagateVarSize=During execution
  Add : Sum
  Add1 : Sum
  Constant7 : Constant  Value=0.0
  Discrete-Time Integrator : DiscreteIntegrator  IntegratorMethod=Integration: Trapezoidal  gainval=Ki  InitialCondition=IC_i  SampleTime=Ts  LimitOutput=on  UpperSaturationLimit=max_i  LowerSaturationLimit=min_i  ICPrevOutput=DiscIntNeverNeededParam  ICPrevScaledInput=DiscIntNeverNeededParam
      settings: AttributesFormatString=Gain=%<gainval>\nMin=%<LowerSaturationLimit>\nMax=%<UpperSaturationLimit>
  Kf : Gain  Gain=Kf
      settings: AttributesFormatString=Gain=%<Gain>
  Saturation : Saturate  UpperLimit=max_out  LowerLimit=min_out
      settings: AttributesFormatString=Min=%<LowerLimit>\nMax=%<UpperLimit>
  Subtract : Sum  Inputs=+-
  Sum2 : Sum  Inputs=|+-  SaturateOnIntegerOverflow=on
  Switch : Switch  Criteria=u2 > Threshold  InputSameDT=off
  Unit Delay : UnitDelay  SampleTime=Ts_Control  HasFrameUpgradeWarning=on
      settings: AttributesFormatString=IC=%<InitialCondition>
  Out : Outport  VectorParamsAs1DForOutWhenUnconnected=off
  wires:
  Kf/1 -> Unit Delay/1
  Subtract/1 -> Switch/3
  Meas/1 -> Subtract/2
  Switch/1 -> Add/1
  Constant7/1 -> Switch/1
  freeze/1 -> Switch/2
  Discrete-Time Integrator/1 -> Add1/2
  Add1/1 -> Sum2/2, Saturation/1
  Sum2/1 -> Kf/1
  Ord/1 -> Subtract/1, Add1/1
  Add/1 -> Discrete-Time Integrator/1
  Unit Delay/1 -> Add/2
  Saturation/1 -> Sum2/1, Out/1

== system ModifiedHVDC/VSC Controller Station 2/Discrete VSC Controller /Outer Active-Reactive Power and Voltage Loop/Active_Power_Control/Ramping ==
  note: Output is reset to zero when the ramp is not enabled
  note: Ramping
  enable_ramp : Inport
  Pref : Inport  Port=2
  Constant12 : Constant  Value=Ramp_apc
  Logical Operator7 : Logic  Operator=NOT  AllPortsSameDT=off
  Rate Limiter with external rates & reset (discrete) IC:0 : Subsystem  mask(Rate of Change Limiter){ic=0, st=Ts_Control}
      mask prompts: ic "Initial condition (pu):"; st "Sample time (s):"
      mask help: Limit rising and falling rates of signal. When the input (R) is true the output is reset to the input (In). Rates are in p.u./s for up and -p.u./s for down.
      mask Display: disp('                Rate\n               Limiter')
  Switch : Switch  Criteria=u2 > Threshold  InputSameDT=off
  zero : Constant  Value=0.0
  Pref_ramp : Outport  VectorParamsAs1DForOutWhenUnconnected=off
  wires:
  Logical Operator7/1 -> Rate Limiter with external rates & reset (discrete) IC:0/4(R)
  Switch/1 -> Rate Limiter with external rates & reset (discrete) IC:0/1(In)
  zero/1 -> Switch/3
  Pref/1 -> Switch/1
  enable_ramp/1 -> Logical Operator7/1, Switch/2
  Constant12/1 -> Rate Limiter with external rates & reset (discrete) IC:0/3(down_rate), Rate Limiter with external rates & reset (discrete) IC:0/2(up_rate)
  Rate Limiter with external rates & reset (discrete) IC:0/1(" ") -> Pref_ramp/1

== system ModifiedHVDC/VSC Controller Station 2/Discrete VSC Controller /Outer Active-Reactive Power and Voltage Loop/Current_Reference_Limitation/Double click here for  info ==
  note: Power System Simulation laboratory (IREQ)
  note: Current Reference Limitation
  note: The subsystem limits the amplitude of phase current of the fundamental component to the rated current
      | of the converter.
  note: Power Control Mode
  note: DC Voltage Control Mode
  note: In power control mode, equal scaling is applied to the active and reactive power reference when a limit is imposed.
  note: In DC voltage control mode, higher priority is given to the active power when a limit is imposed.

== system ModifiedHVDC/VSC Controller Station 2/Discrete VSC Controller /Outer Active-Reactive Power and Voltage Loop/DC_Voltage_Control/PI_regulator (type 2) ==
  note: Regulator PI
      | (Type 2)
  Ord : Inport
  Meas : Inport  Port=2
  Add : Sum
  Add1 : Sum
  Discrete-Time Integrator : DiscreteIntegrator  IntegratorMethod=Integration: Trapezoidal  gainval=Ki  InitialCondition=i_ic  SampleTime=Ts  LimitOutput=on  UpperSaturationLimit=max_i  LowerSaturationLimit=min_i  ICPrevOutput=DiscIntNeverNeededParam  ICPrevScaledInput=DiscIntNeverNeededParam
      settings: AttributesFormatString=Gain=%<gainval>\nMin=%<LowerSaturationLimit>\nMax=%<UpperSaturationLimit>
  Kf : Gain  Gain=Kf
      settings: AttributesFormatString=Gain=%<Gain>
  Kp : Gain  Gain=Kp
      settings: AttributesFormatString=Gain=%<Gain>
  Saturation : Saturate  UpperLimit=max_out  LowerLimit=min_out
      settings: AttributesFormatString=Min=%<LowerLimit>\nMax=%<UpperLimit>
  Subtract : Sum  Inputs=+-
  Sum2 : Sum  Inputs=|+-  SaturateOnIntegerOverflow=on
  Unit Delay : UnitDelay  SampleTime=Ts_Control  HasFrameUpgradeWarning=on
      settings: AttributesFormatString=IC=%<InitialCondition>
  Out : Outport  VectorParamsAs1DForOutWhenUnconnected=off
  wires:
  Kp/1 -> Add1/1
  Sum2/1 -> Kf/1
  Subtract/1 -> Add/1, Kp/1
  Saturation/1 -> Sum2/1, Out/1
  Unit Delay/1 -> Add/2
  Add/1 -> Discrete-Time Integrator/1
  Ord/1 -> Subtract/1
  Kf/1 -> Unit Delay/1
  Add1/1 -> Saturation/1, Sum2/2
  Discrete-Time Integrator/1 -> Add1/2
  Meas/1 -> Subtract/2
